simulink model "main_sim_mk15_pi"  (R2024b)
settings: Solver=ode23t  StartTime=0.0  StopTime=0.9  MaxStep=1e-7  RelTol=0.5e-5
InitFcn:
  | sw_freq=50e3;
  | kp=0.035;
  | ki=3.2;
libraries: spsSeriesRLCBranchLib x24, spsMeanLib x13, spsCurrentMeasurementLib x7, spsVoltageMeasurementLib x6, spsDiodeLib x6, spsControlledCurrentSourceLib x5, spsControlledVoltageSourceLib x5, spsMosfetLib x4, spsIdealSwitchLib x4, eeStairGenerator x2, embmathops x1, spsGroundLib x1
settings Model: SimulationMode=rapid-accelerator  Creator=adamo  LastModifiedBy=adamo
settings SolverCC: AllowMultiTaskInputOutput=on  ZeroCrossAlgorithm=Adaptive  SolverResetMethod=Robust  PositivePriorityOrder=on  DecoupledContinuousIntegration=on  MinimalZcImpactIntegration=on
settings OptimizationCC: ReuseModelBlockBuffer=off  SimCompilerOptimization=on
settings DebuggingCC: AlgebraicLoopMsg=none  MaskedZcDiagnostic=none  IgnoredZcDiagnostic=none
settings HardwareCC: ProdHWDeviceType=AMD->x86-64 (Windows64)
settings ModelReferenceCC: EnableParallelModelReferenceBuilds=on  ParallelModelReferenceMATLABWorkerInit=Copy Base Workspace  ModelReferenceMinAlgLoopOccurrences=on
settings SFSimCC: SimHardwareAcceleration=native  SimTargetLang=C++
settings RTWCC: BuildConfiguration=Faster Runs  GPUComputeCapability=3.5
settings GRTTargetCC: OptimizeReductions=on

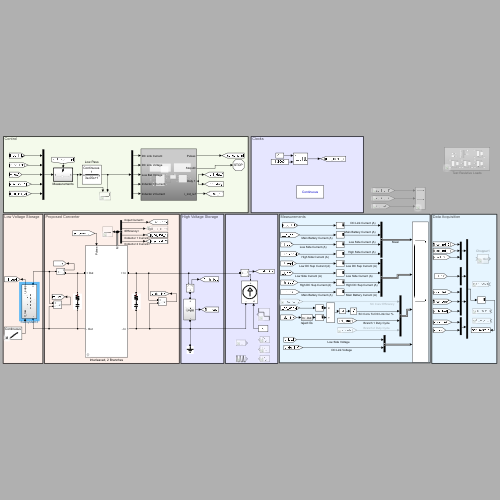
[thumbnail: Simulink's stored preview of the top-level diagram]
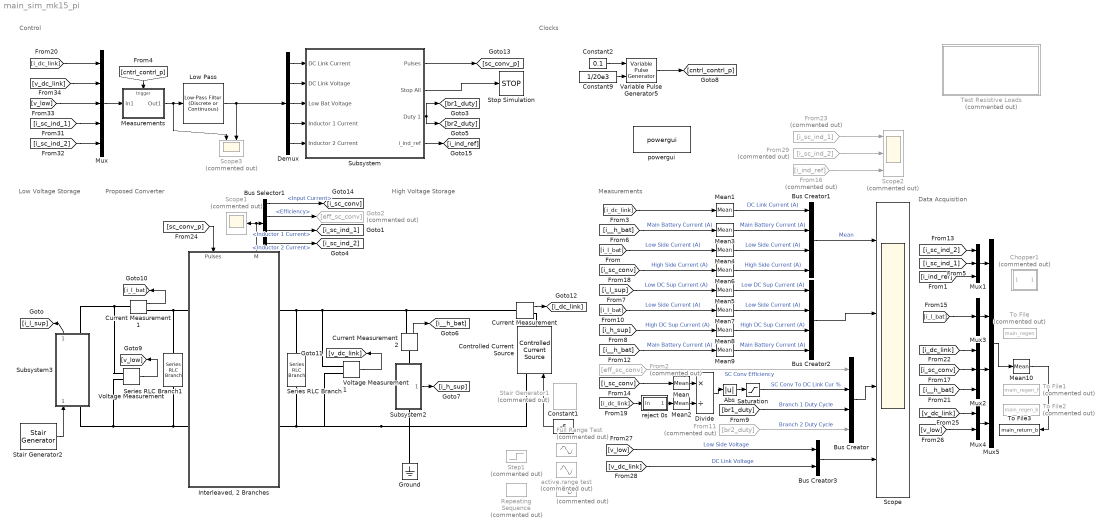
== system main_sim_mk15_pi ==
  note: Data Acquisition
  note: High Voltage Storage
  note: Low Voltage Storage
  note: Proposed Converter
  note: Clocks
  note: Control
  note: Measurements
  " " : Sin  Commented=on  Amplitude=8  Bias=18  Frequency=314.1592/10  SampleTime=0
  Abs : Abs  SaturateOnIntegerOverflow=off
  Bus Creator : BusCreator  Inputs=4
  Bus Creator1 : BusCreator  Inputs=4
  Bus Creator2 : BusCreator  Inputs=4
  Bus Creator3 : BusCreator  Inputs=2
  Bus Selector1 : BusSelector  OutputSignals=Input Current,Efficiency,Inductor 1 Current,Inductor 2 Current
  Chopper1 : Subsystem  Commented=on
  Constant1 : Constant  Value=-6
  Constant2 : Constant  Value=0.1
  Constant9 : Constant  Value=1/20e3
  Controlled Current Source : spsControlledCurrentSourceLib/Controlled Current Source  Initialize=on  Source_Type=DC  Amplitude=0  Phase=0  Frequency=0  Measurements=None
  Current Measurement : spsCurrentMeasurementLib/Current Measurement  PhasorSimulation=off  OutputType=Complex  PSBequivalent=0
  Current Measurement1 : spsCurrentMeasurementLib/Current Measurement  PhasorSimulation=off  OutputType=Complex  PSBequivalent=0
  Current Measurement2 : spsCurrentMeasurementLib/Current Measurement  PhasorSimulation=off  OutputType=Complex  PSBequivalent=0
  Demux : Demux  Outputs=5
  Divide : Product  Inputs=*/
  From11 : From  Commented=on  GotoTag=br2_duty
  From16 : From  Commented=on  GotoTag=i_ind_ref
  From2 : From  Commented=on  GotoTag=eff_sc_conv
  From23 : From  Commented=on  GotoTag=i_sc_ind_1
  From29 : From  Commented=on  GotoTag=i_sc_ind_2
  Full Range Test : Sin  Commented=on  Amplitude=52  Frequency=314.1592/8  SampleTime=0
  Goto2 : Goto  Commented=on  GotoTag=eff_sc_conv
  Ground : spsGroundLib/Ground  LConnTagsString=a
  "Interleaved, 2 Branches" : Subsystem  mask{sw_freq_mean=sw_freq, ind_ind=200e-6, fet_res_on=10e-3, bd_d_for_volt=1.1}
      mask prompts: sw_freq_mean "Switching Frequency (Hz)"; ind_ind "Branch Inductor Inductance (H)"; fet_res_on "Drain-to-Source On-Resistance (Ohm)"; bd_d_for_volt "Body Diode Forward Voltage (V)"
      settings: PortSchema="{\"entries\":[{\"content\":{\"sides\":[{\"content\":{\"connectorIds\":[\"LConn1\",\"LConn2\"]},\"type\":\"ConnectorPlacement.EquallySpacedRectSide\",\"uuid\":\"57763a22-817d-4d04-a19a-6b084199baa7\"},{\"content\":{\"connectorIds\":[\"RConn1\",\"RConn2\"],\"side\":\"RIGHT\"},\"type\":\"ConnectorPlacement.EquallySpacedRectSide\",\"uuid\":\"e5f04f53-fac9-409a-ac58-f518a07f7aa1\"},{\"content\":{\"connectorIds\":[\"In1\",\"Out1\"],\"side\":\"TOP\"},\"type\":\"ConnectorPlacement.EquallySpacedRectSide\",\"uuid\":\"7683f119-33ed-4468-84c8-2aaaca937041\"}]},\"type\":\"ConnectorPlacement.EquallySpacedConnector\",\"uuid\":\"94c2a178-e796-4540-a87e-c79e0224e730\"}],\"packageUris\":[\"http://schema.mathworks.com/mf0/Connector/R2020b\"],\"version\":\"1.0\"}"
      mask DialogControl DescTextVar Prompt: %<MaskDescription>This block impements a Two Phase Interleaved Bidirectional DC-DC Buck/Boost Converter. Input is the left side (High Voltage Side). All MOSFETs share the same characteristics.
      mask DialogControl ParameterGroupVar Prompt: Circuit Parameters
      mask DialogControl Container3 Prompt: MOSFET Parameters
  Low Pass : eeGeneralControl/Low-Pass Filter (Discrete or Continuous)  K=1  T=0.00003  B=150  A=-150  init_option=Inherited from block input  x0=0  Ts=0
  Mean : spsMeanLib/Mean  Freq=50e3/100  Vinit=0  Ts=0
  Mean{1,3..9} (8 alike) : spsMeanLib/Mean  Freq=50e3/50  Vinit=0  Ts=0
  Mean10 : spsMeanLib/Mean  Freq=50e3/100  Vinit=0  Ts=0
  Mean2 : spsMeanLib/Mean  Freq=50e3/100  Vinit=0  Ts=0
  Measurements : Subsystem  TreatAsAtomicUnit=on
  Mux : Mux  Inputs=5
  Mux1 : Mux  Inputs=3
  Mux2 : Mux  Inputs=3
  Mux3 : Mux  Inputs=1
  Mux4 : Mux  Inputs=2
  Mux5 : Mux
  Repeating Sequence : simulink/Sources/Repeating Sequence  Commented=on  rep_seq_t=[0 0.5 1 2]*2  rep_seq_y=[0 16 0 0]
  Saturation : Saturate  UpperLimit=1  LowerLimit=0
  Scope : Scope  NumInputPorts=4
  Scope1 : Scope  Commented=on
  Scope2 : Scope  Commented=on  NumInputPorts=3
  Scope3 : Scope  Commented=on  NumInputPorts=2
  Series RLC Branch : spsSeriesRLCBranchLib/Series RLC Branch  LConnTagsString=__new0  RConnTagsString=__new0  BranchType=RC  Resistance=1e-4  Inductance=1e-3  SetiL0=off  InitialCurrent=0  Capacitance=800e-6  Setx0=on  InitialVoltage=80  Measurements=None
  Series RLC Branch1 : spsSeriesRLCBranchLib/Series RLC Branch  LConnTagsString=__new0  RConnTagsString=__new0  BranchType=RC  Resistance=1e-4  Inductance=1e-3  SetiL0=off  InitialCurrent=0  Capacitance=400e-6  Setx0=on  InitialVoltage=15  Measurements=None
  Stair Generator1 : spsStairGeneratorLib/Stair Generator  Commented=on  t=[0:1:3]  e=[12.5:-2.5:5]  Ts=0
  Stair Generator2 : eeStairGenerator/Stair Generator  LabelModeActiveChoice=Continuous  TimeInput=[0:0.15:1]  AmplitudeInput=[15:5:45]  SampleTime=0  RepeatPattern=off  OutDataTypeStr=double
      settings: LibrarySourceBlock=ee_sl_lib/General Control/Stair Generator
  Step1 : Step  Commented=on  Time=0.1  Before=27  After=-25  SampleTime=0
  Stop Simulation : Stop
  Subsystem : Subsystem
  Subsystem2 : Subsystem
      settings: PortSchema="{\"entries\":[{\"content\":{\"sides\":[{\"content\":{},\"type\":\"ConnectorPlacement.EquallySpacedRectSide\",\"uuid\":\"89586188-a7fa-42d8-902c-41f5e85746df\"},{\"content\":{\"connectorIds\":[\"Out1\"],\"side\":\"RIGHT\"},\"type\":\"ConnectorPlacement.EquallySpacedRectSide\",\"uuid\":\"d8c02237-7822-43ca-9dbf-595cafdf61ba\"},{\"content\":{\"connectorIds\":[\"LConn1\"],\"side\":\"TOP\"},\"type\":\"ConnectorPlacement.EquallySpacedRectSide\",\"uuid\":\"69757e4c-b908-4056-b98e-0c667e12b99a\"},{\"content\":{\"connectorIds\":[\"RConn1\"],\"side\":\"BOTTOM\"},\"type\":\"ConnectorPlacement.EquallySpacedRectSide\",\"uuid\":\"ccf2e3d8-e338-404e-98cd-f765717e085e\"}]},\"type\":\"ConnectorPlacement.EquallySpacedConnector\",\"uuid\":\"a290fee4-a270-4f54-b8a3-7452b5039597\"}],\"packageUris\":[\"http://schema.mathworks.com/mf0/Connector/R2020b\"],\"version\":\"1.0\"}"
  Subsystem3 : Subsystem
      settings: PortSchema="{\"entries\":[{\"content\":{\"sides\":[{\"content\":{},\"type\":\"ConnectorPlacement.EquallySpacedRectSide\",\"uuid\":\"89586188-a7fa-42d8-902c-41f5e85746df\"},{\"content\":{\"side\":\"RIGHT\"},\"type\":\"ConnectorPlacement.EquallySpacedRectSide\",\"uuid\":\"d8c02237-7822-43ca-9dbf-595cafdf61ba\"},{\"content\":{\"connectorIds\":[\"LConn1\",\"Out1\"],\"side\":\"TOP\"},\"type\":\"ConnectorPlacement.EquallySpacedRectSide\",\"uuid\":\"69757e4c-b908-4056-b98e-0c667e12b99a\"},{\"content\":{\"connectorIds\":[\"RConn1\",\"In1\"],\"side\":\"BOTTOM\"},\"type\":\"ConnectorPlacement.EquallySpacedRectSide\",\"uuid\":\"e30ca493-d5d4-4c79-9ea0-2752edd701ef\"}]},\"type\":\"ConnectorPlacement.EquallySpacedConnector\",\"uuid\":\"a290fee4-a270-4f54-b8a3-7452b5039597\"}],\"packageUris\":[\"http://schema.mathworks.com/mf0/Connector/R2020b\"],\"version\":\"1.0\"}"
  Test Resistive Loads : Subsystem  Commented=on
  To File : ToFile  Commented=on  Filename=main_regen
  To File1 : ToFile  Commented=on  Filename=main_regen_f
  To File2 : ToFile  Commented=on  Filename=main_regen_b
  To File3 : ToFile  Filename=main_return_b
  Variable Pulse Generator5 : VariablePulseGenerator  AllowZeroPulseWidth=on  SampleTime=0.1
  Voltage Measurement : spsVoltageMeasurementLib/Voltage Measurement  PhasorSimulation=off  OutputType=Complex  PSBequivalent=0
  Voltage Measurement1 : spsVoltageMeasurementLib/Voltage Measurement  PhasorSimulation=off  OutputType=Complex  PSBequivalent=0
  active range test : Sin  Commented=on  Amplitude=24  Bias=4  Frequency=314.1592/32  SampleTime=0
  powergui : spspowerguiLib/powergui  Priority=1  SimulationMode=Continuous  SampleTime=50e-6  frequency=60  Iterations=50  frequencyindice=0  Pbase=100e6  ErrMax=1e-4  UnitsV=kV  UnitsW=MW  buscounter=0  FunctionMessages=off  echomessages=off  EnableUseOfTLC=off  CurrentSourceSwitches=off  DisableSnubberDevices=on  DisableRonSwitches=off  DisableVfSwitches=off  DisplayEquations=off  AutomaticDiscreteSolvers=off  SolverType=Tustin/Backward Euler (TBE)  Interpol=off  ExternalGateDelay=off  methode=off  Ts=100  x0status=blocks  SPID=on  SwTol=0  HookPort=off  NonlinearTolerance=1e-4  nMaxIteration=100  ContinueOnMaxIteration=off  RestoreLinks=warning  ResistiveCurrentMeasurement=off  Frange=[0:2:500]  Ylog=off  Xlog=on  ShowGrid=off  save=off  variable=ZData  structure=0  ZoomFFT=off  StartTime=0.0  cycles=1  DisplayStyle=1  fundamental=60  FreqAxis=off  MaxFrequency=1000  frequencyindicesteady=1  RmsSteady=1  display=off
  reject 0s : Subsystem
  wires:
  Bus Creator2/1 -> Scope/2
  Mean3/1 -> Bus Creator1/2  "Main Battery Current (A)"
  Mean4/1 -> Bus Creator1/3  "Low Side Current (A)"
  Bus Selector1/2 -> Goto2/1  "<Efficiency>"
  From2/1 -> Bus Creator/1  "SC Conv Efficiency"
  Bus Selector1/1 -> [i_sc_conv]  "<Input Current>"
  reject 0s/1(Out) -> Mean2/1
  Divide/1 -> Abs/1
  Abs/1 -> Saturation/1
  [i_sc_conv] -> Mean/1
  Saturation/1 -> Bus Creator/2  "SC Conv To DC Link Cur %"
  [i_dc_link] -> reject 0s/1(In)
  Bus Creator/1 -> Scope/3
  Bus Creator1/1 -> Scope/1  "Mean"
  Mean/1 -> Divide/1
  Mean2/1 -> Divide/2
  Mean1/1 -> Bus Creator1/1  "DC Link Current (A)"
  [i__h_bat] -> Mean3/1  "Main Battery Current (A)"
  [i_l_bat] -> Mean4/1  "Low Side Current (A)"
  Mean6/1 -> Bus Creator1/4  "High Side Current (A)"
  [i_sc_conv] -> Mean6/1  "High Side Current (A)"
  [sc_conv_p] -> "Interleaved, 2 Branches"/1(Pulses)
  Subsystem2/1(i_supp) -> [i_h_sup]
  [i_dc_link] -> Mean1/1
  Current Measurement/1 -> [i_dc_link]
  Bus Selector1/3 -> [i_sc_ind_1]  "<Inductor 1 Current>"
  Bus Selector1/4 -> [i_sc_ind_2]  "<Inductor 2 Current>"
  Voltage Measurement/1 -> [v_low]
  Current Measurement1/1 -> [i_l_bat]
  Constant2/1 -> Variable Pulse Generator5/1
  Constant9/1 -> Variable Pulse Generator5/2
  Variable Pulse Generator5/1 -> [cntrl_contrl_p]
  Subsystem/1(Pulses) -> [sc_conv_p]
  [i_sc_ind_2] -> Mux/5
  [i_sc_ind_1] -> Mux/4
  [v_low] -> Mux/3
  [v_dc_link] -> Mux/2
  [i_dc_link] -> Mux/1
  Demux/1 -> Subsystem/1(DC Link Current)
  Demux/2 -> Subsystem/2(DC Link Voltage)
  Demux/3 -> Subsystem/3(Low Bat Voltage)
  Demux/5 -> Subsystem/5(Inductor 2 Current)
  Demux/4 -> Subsystem/4(Inductor 1 Current)
  [cntrl_contrl_p] -> Measurements/Trigger
  Subsystem/2(Stop All) -> Stop Simulation/1
  Subsystem/3(Duty 1) -> [br1_duty], [br2_duty]
  From11/1 -> Bus Creator/4  "Branch 2 Duty Cycle"
  [br1_duty] -> Bus Creator/3  "Branch 1 Duty Cycle"
  Bus Creator3/1 -> Scope/4
  Current Measurement2/1 -> [i__h_bat]
  Subsystem3/1(i_supp) -> [i_l_sup]
  Mean5/1 -> Bus Creator2/1  "Low DC Sup Current (A)"
  Mean7/1 -> Bus Creator2/2  "Low Side Current (A)"
  Mean8/1 -> Bus Creator2/3  "High DC Sup Current (A)"
  Mean9/1 -> Bus Creator2/4  "Main Battery Current (A)"
  [i_l_sup] -> Mean5/1  "Low DC Sup Current (A)"
  [i_l_bat] -> Mean7/1  "Low Side Current (A)"
  [i_h_sup] -> Mean8/1  "High DC Sup Current (A)"
  [i__h_bat] -> Mean9/1  "Main Battery Current (A)"
  Voltage Measurement1/1 -> [v_dc_link]
  Mux/1 -> Measurements/1(In1)
  Measurements/1(Out1) -> Scope3/1, Low Pass/1
  Subsystem/4(i_ind_ref) -> [i_ind_ref]
  [i_sc_ind_2] -> Mux1/1
  [i_sc_ind_1] -> Mux1/2
  [i_ind_ref] -> Mux1/3
  [i_dc_link] -> Mux2/1
  [i_sc_conv] -> Mux2/2
  [i__h_bat] -> Mux2/3
  [i_l_bat] -> Mux3/1
  [v_low] -> Mux4/2
  [v_dc_link] -> Mux4/1
  Mux1/1 -> Mux5/1
  Mux3/1 -> Mux5/2
  Mux2/1 -> Mux5/3
  Mux4/1 -> Mux5/4
  Mux5/1 -> Mean10/1
  Stair Generator2/1 -> Subsystem3/1(V_low)
  [v_low] -> Bus Creator3/1  "Low Side Voltage"
  [v_dc_link] -> Bus Creator3/2  "DC Link Voltage"
  "Interleaved, 2 Branches"/1(M) -> Scope1/1, Bus Selector1/1
  Low Pass/1 -> Demux/1, Scope3/2
  Constant1/1 -> Controlled Current Source/1
  Mean10/1 -> To File3/1
  From23/1 -> Scope2/1
  From16/1 -> Scope2/3
  From29/1 -> Scope2/2
  connections:
  Series RLC Branch/RConn1 -- Voltage Measurement1/LConn2 -- Controlled Current Source/LConn1 -- Ground/LConn1 -- Subsystem2/RConn1 -- "Interleaved, 2 Branches"/RConn2
  "Interleaved, 2 Branches"/LConn2 -- Series RLC Branch1/RConn1 -- Subsystem3/RConn1 -- Voltage Measurement/LConn2
  Controlled Current Source/RConn1 -- Current Measurement/RConn1
  Voltage Measurement/LConn1 -- Subsystem3/LConn1 -- Current Measurement1/LConn1
  Current Measurement/LConn1 -- Current Measurement2/RConn1 -- Voltage Measurement1/LConn1 -- "Interleaved, 2 Branches"/RConn1 -- Series RLC Branch/LConn1
  "Interleaved, 2 Branches"/LConn1 -- Series RLC Branch1/LConn1 -- Current Measurement1/RConn1
  Current Measurement2/LConn1 -- Subsystem2/LConn1

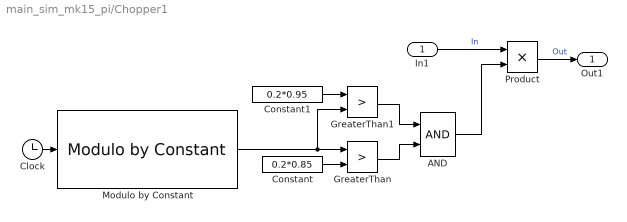
== system main_sim_mk15_pi/Chopper1 ==
  In1 : Inport
  AND : Logic  IconShape=distinctive  AllPortsSameDT=off  OutDataTypeStr=boolean
  Clock : Clock
  Constant : Constant  Value=0.2*0.85
  Constant1 : Constant  Value=0.2*0.95
  GreaterThan : RelationalOperator  Operator=>  OutDataTypeStr=boolean  RndMeth=Simplest  InputSameDT=off
  GreaterThan1 : RelationalOperator  Operator=>  OutDataTypeStr=boolean  RndMeth=Simplest  InputSameDT=off
  Modulo by Constant : embmathops/Modulo by Constant  Denominator=0.2  SimulateUsing=Code generation
  Product : Product
  Out1 : Outport
  wires:
  Clock/1 -> Modulo by Constant/1
  Constant/1 -> GreaterThan/2
  GreaterThan1/1 -> AND/1
  GreaterThan/1 -> AND/2
  AND/1 -> Product/2
  Modulo by Constant/1 -> GreaterThan1/2, GreaterThan/1
  Constant1/1 -> GreaterThan1/1
  In1/1 -> Product/1  "In"
  Product/1 -> Out1/1  "Out"

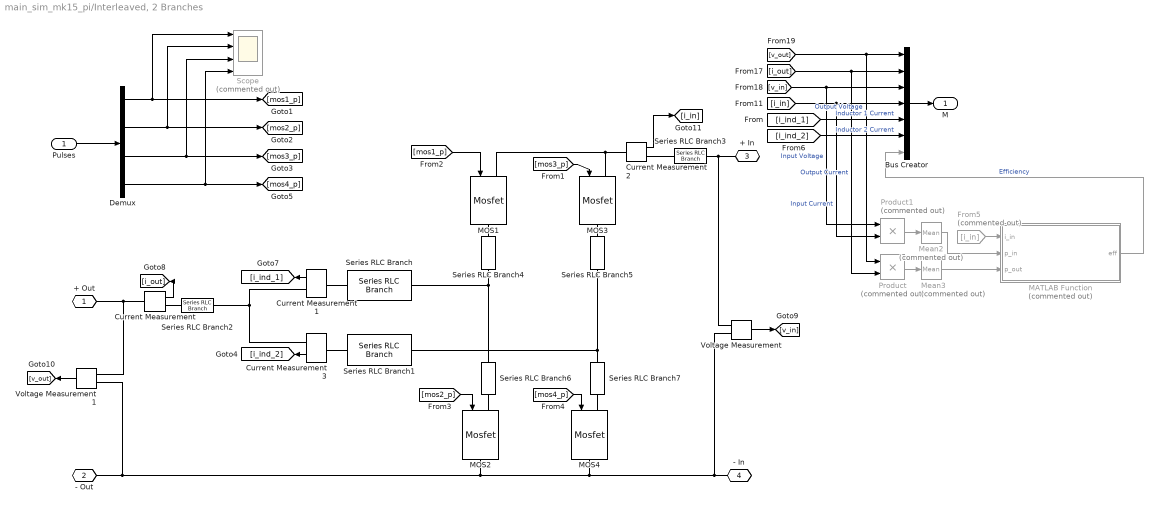
== system main_sim_mk15_pi/Interleaved, 2 Branches ==
  Pulses : Inport
  Bus Creator : BusCreator  Inputs=7
  Current Measurement{,1..3} (4 alike) : spsCurrentMeasurementLib/Current Measurement  PhasorSimulation=off  OutputType=Complex  PSBequivalent=0
  Demux : Demux
  From5 : From  Commented=on  GotoTag=i_in
  MATLAB Function : MATLAB Function  Commented=on  TreatAsAtomicUnit=on
  MOS{1..4} (4 alike) : spsMosfetLib/Mosfet  Ron=fet_res_on  Lon=0  Rd=0.01  Vfd=bd_d_for_volt  IC=0  Rs=1e5  Cs=inf  Measurements=off
  Mean2 : spsMeanLib/Mean  Commented=on  Freq=sw_freq_mean/10  Vinit=0  Ts=0
  Mean3 : spsMeanLib/Mean  Commented=on  Freq=sw_freq_mean/10  Vinit=0  Ts=0
  Product : Product  Commented=on
  Product1 : Product  Commented=on
  Scope : Scope  Commented=on  NumInputPorts=4
  Series RLC Branch : spsSeriesRLCBranchLib/Series RLC Branch  LConnTagsString=__new0  RConnTagsString=__new0  BranchType=RL  Resistance=1e-3  Inductance=ind_ind  SetiL0=off  InitialCurrent=1e-3  Capacitance=1e-6  Setx0=off  InitialVoltage=0  Measurements=None
  Series RLC Branch1 : spsSeriesRLCBranchLib/Series RLC Branch  LConnTagsString=__new0  RConnTagsString=__new0  BranchType=RL  Resistance=1e-3  Inductance=ind_ind  SetiL0=off  InitialCurrent=1e-3  Capacitance=1e-6  Setx0=off  InitialVoltage=0  Measurements=None
  Series RLC Branch2 : spsSeriesRLCBranchLib/Series RLC Branch  LConnTagsString=__new0  RConnTagsString=__new0  BranchType=R  Resistance=5e-3  Inductance=5e-4  SetiL0=off  InitialCurrent=1e-3  Capacitance=1e-6  Setx0=off  InitialVoltage=0  Measurements=None
  Series RLC Branch3 : spsSeriesRLCBranchLib/Series RLC Branch  LConnTagsString=__new0  RConnTagsString=__new0  BranchType=R  Resistance=5e-3  Inductance=5e-4  SetiL0=off  InitialCurrent=1e-3  Capacitance=1e-6  Setx0=off  InitialVoltage=0  Measurements=None
  Series RLC Branch{4..7} (4 alike) : spsSeriesRLCBranchLib/Series RLC Branch  LConnTagsString=__new0  RConnTagsString=__new0  BranchType=R  Resistance=1e-3  Inductance=5e-4  SetiL0=off  InitialCurrent=1e-3  Capacitance=1e-6  Setx0=off  InitialVoltage=0  Measurements=None
  Voltage Measurement : spsVoltageMeasurementLib/Voltage Measurement  PhasorSimulation=off  OutputType=Complex  PSBequivalent=0
  Voltage Measurement1 : spsVoltageMeasurementLib/Voltage Measurement  PhasorSimulation=off  OutputType=Complex  PSBequivalent=0
  + Out : PMIOPort  Side=Left
  - Out : PMIOPort  Port=2  Side=Left
  "+ In " : PMIOPort  Port=3  Side=Right
  "- In " : PMIOPort  Port=4  Side=Right
  M : Outport
  wires:
  [mos1_p] -> MOS1/1
  [mos2_p] -> MOS2/1
  Current Measurement1/1 -> [i_ind_1]
  Current Measurement2/1 -> [i_in]
  Voltage Measurement1/1 -> [v_out]
  Voltage Measurement/1 -> [v_in]
  [i_ind_2] -> Bus Creator/6  "Inductor 2 Current"
  Bus Creator/1 -> M/1
  [v_in] -> Bus Creator/3, Product1/1  "Input Voltage"
  [i_out] -> Product/2, Bus Creator/2  "Output Current"
  [i_in] -> Product1/2, Bus Creator/4  "Input Current"
  [v_out] -> Product/1, Bus Creator/1  "Output Voltage"
  MATLAB Function/1(eff) -> Bus Creator/7  "Efficiency"
  Product/1 -> Mean3/1
  Product1/1 -> Mean2/1
  From5/1 -> MATLAB Function/1(i_in)
  Pulses/1 -> Demux/1
  Demux/1 -> Scope/1, [mos1_p]
  Mean2/1 -> MATLAB Function/2(p_in)
  Mean3/1 -> MATLAB Function/3(p_out)
  Current Measurement/1 -> [i_out]
  [mos3_p] -> MOS3/1
  Current Measurement3/1 -> [i_ind_2]
  [i_ind_1] -> Bus Creator/5  "Inductor 1 Current"
  Demux/3 -> Scope/3, [mos3_p]
  Demux/4 -> Scope/4, [mos4_p]
  Demux/2 -> Scope/2, [mos2_p]
  [mos4_p] -> MOS4/1
  connections:
  MOS1/LConn1 -- Current Measurement2/LConn1 -- MOS3/LConn1
  Voltage Measurement1/LConn1 -- Current Measurement/LConn1 -- + Out/RConn1
  "+ In "/RConn1 -- Voltage Measurement/LConn1 -- Series RLC Branch3/RConn1
  "- In "/RConn1 -- Voltage Measurement/LConn2 -- Voltage Measurement1/LConn2 -- - Out/RConn1 -- MOS2/RConn1 -- MOS4/RConn1
  Series RLC Branch/LConn1 -- Current Measurement1/LConn1
  Series RLC Branch/RConn1 -- Series RLC Branch6/LConn1 -- Series RLC Branch4/RConn1
  Series RLC Branch1/RConn1 -- Series RLC Branch7/LConn1 -- Series RLC Branch5/RConn1
  Series RLC Branch1/LConn1 -- Current Measurement3/LConn1
  Series RLC Branch2/RConn1 -- Current Measurement3/RConn1 -- Current Measurement1/RConn1
  Series RLC Branch2/LConn1 -- Current Measurement/RConn1
  Series RLC Branch4/LConn1 -- MOS1/RConn1
  Series RLC Branch5/LConn1 -- MOS3/RConn1
  Series RLC Branch6/RConn1 -- MOS2/LConn1
  Series RLC Branch7/RConn1 -- MOS4/LConn1
  Series RLC Branch3/LConn1 -- Current Measurement2/RConn1

== system main_sim_mk15_pi/Measurements ==
  In1 : Inport
  Trigger : TriggerPort  VariantControl=(inherit)
  Zero-Order Hold : ZeroOrderHold  SampleTime=-1
  Out1 : Outport
  wires:
  In1/1 -> Zero-Order Hold/1
  Zero-Order Hold/1 -> Out1/1

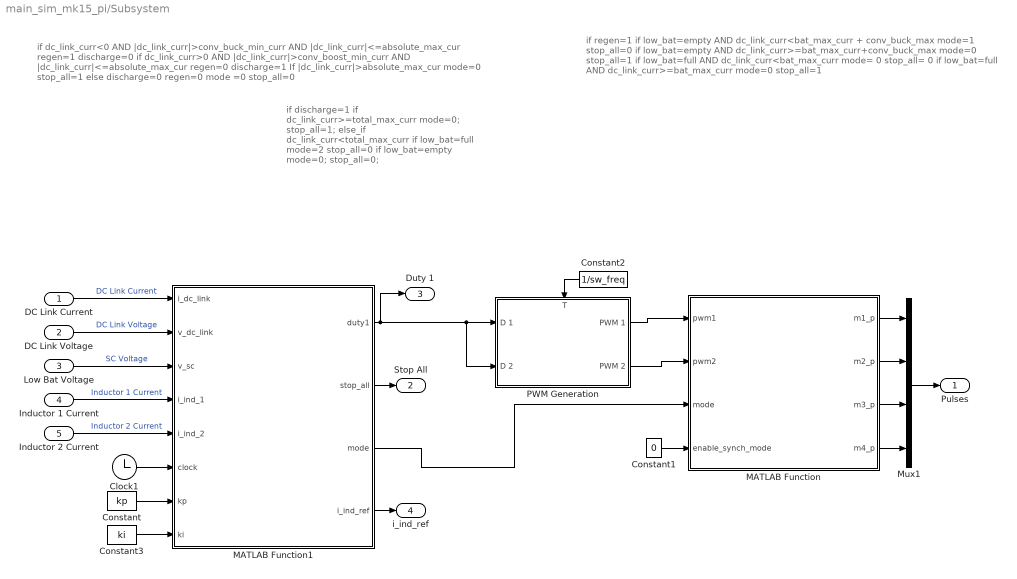
== system main_sim_mk15_pi/Subsystem ==
  note: if regen=1
      | 	if low_bat=empty AND dc_link_curr<bat_max_curr + conv_buck_max
      | 		mode=1
      | 		stop_all=0
      | 	if low_bat=empty AND dc_link_curr>=bat_max_curr+conv_buck_max
      | 		mode=0
      | 		stop_all=1
      | 	if low_bat=full AND dc_link_curr<bat_max_curr
      | 		mode= 0
      | 		stop_all= 0
      | 	if low_bat=full AND dc_link_curr>=bat_max_curr
      | 		mode=0
      | 		stop_all=1
  note: if discharge=1
      | 	if dc_link_curr>=total_max_curr
      | 		mode=0;
      | 		stop_all=1;
      | 	else_if dc_link_curr<total_max_curr
      | 		if low_bat=full
      | 			mode=2
      | 			stop_all=0
      | 		if low_bat=empty
      | 			mode=0;
      | 			stop_all=0;
  note: if dc_link_curr<0 AND |dc_link_curr|>conv_buck_min_curr AND |dc_link_curr|<=absolute_max_cur
      | 	regen=1
      | 	discharge=0
      | if dc_link_curr>0 AND |dc_link_curr|>conv_boost_min_curr AND |dc_link_curr|<=absolute_max_cur
      | 	regen=0
      | 	discharge=1
      | If  |dc_link_curr|>absolute_max_cur
      | 	mode=0
      | 	stop_all=1
      | else
      | 	discharge=0
      | 	regen=0
      | 	mode =0
      | 	stop_all=0
  DC Link Current : Inport
  DC Link Voltage : Inport  Port=2
  Low Bat Voltage : Inport  Port=3
  Inductor 1 Current : Inport  Port=4
  Inductor 2 Current : Inport  Port=5
  Clock1 : Clock
      settings: Decimation=20
  Constant : Constant  Value=kp
  Constant1 : Constant  Value=0
  Constant2 : Constant  Value=1/sw_freq
  Constant3 : Constant  Value=ki
  MATLAB Function : MATLAB Function  TreatAsAtomicUnit=on
  MATLAB Function1 : MATLAB Function  TreatAsAtomicUnit=on
  Mux1 : Mux
  PWM Generation : Subsystem
      settings: PortSchema="{\"entries\":[{\"content\":{\"sides\":[{\"content\":{\"connectorIds\":[\"In1\",\"In2\"]},\"type\":\"ConnectorPlacement.EquallySpacedRectSide\",\"uuid\":\"83f7ddc5-a76f-4bd9-b3c1-9fd524e2bc79\"},{\"content\":{\"connectorIds\":[\"Out1\",\"Out2\"],\"side\":\"RIGHT\"},\"type\":\"ConnectorPlacement.EquallySpacedRectSide\",\"uuid\":\"761d98eb-d7f1-4fa1-8255-54b7e6584824\"},{\"content\":{\"connectorIds\":[\"In3\"],\"side\":\"TOP\"},\"type\":\"ConnectorPlacement.EquallySpacedRectSide\",\"uuid\":\"fcf92395-65ef-4712-95c3-1cc1de5b2992\"}]},\"type\":\"ConnectorPlacement.EquallySpacedConnector\",\"uuid\":\"c82b4b62-fa36-4445-aa1a-cfaf75c093b5\"}],\"packageUris\":[\"http://schema.mathworks.com/mf0/Connector/R2020b\"],\"version\":\"1.0\"}"
  Pulses : Outport
  Stop All : Outport  Port=2
  Duty 1 : Outport  Port=3
  i_ind_ref : Outport  Port=4
  wires:
  DC Link Voltage/1 -> MATLAB Function1/2(v_dc_link)  "DC Link Voltage"
  DC Link Current/1 -> MATLAB Function1/1(i_dc_link)  "DC Link Current"
  Low Bat Voltage/1 -> MATLAB Function1/3(v_sc)  "SC Voltage"
  Inductor 1 Current/1 -> MATLAB Function1/4(i_ind_1)  "Inductor 1 Current"
  Inductor 2 Current/1 -> MATLAB Function1/5(i_ind_2)  "Inductor 2 Current"
  MATLAB Function1/2(stop_all) -> Stop All/1
  MATLAB Function1/3(mode) -> MATLAB Function/3(mode)
  Mux1/1 -> Pulses/1
  Clock1/1 -> MATLAB Function1/6(clock)
  MATLAB Function/1(m1_p) -> Mux1/1
  MATLAB Function/2(m2_p) -> Mux1/2
  MATLAB Function/3(m3_p) -> Mux1/3
  MATLAB Function/4(m4_p) -> Mux1/4
  Constant1/1 -> MATLAB Function/4(enable_synch_mode)
  MATLAB Function1/1(duty1) -> Duty 1/1, PWM Generation/2(D 2), PWM Generation/1(D 1)
  PWM Generation/1(PWM 1) -> MATLAB Function/1(pwm1)
  PWM Generation/2(PWM 2) -> MATLAB Function/2(pwm2)
  Constant2/1 -> PWM Generation/3(T)
  MATLAB Function1/4(i_ind_ref) -> i_ind_ref/1
  Constant/1 -> MATLAB Function1/7(kp)
  Constant3/1 -> MATLAB Function1/8(ki)

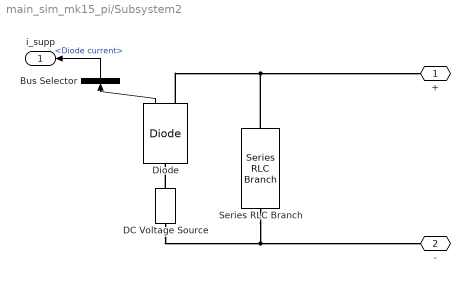
== system main_sim_mk15_pi/Subsystem2 ==
  Bus Selector : BusSelector  OutputSignals=Diode current
  DC Voltage Source : spsDCVoltageSourceLib/DC Voltage Source  Amplitude=80  Measurements=None
  Diode : spsDiodeLib/Diode  Ron=0.001  Lon=0  Vf=0.01  IC=0  UseSnubber=0  Rs=500  Cs=250e-9  Measurements=on
  Series RLC Branch : spsSeriesRLCBranchLib/Series RLC Branch  LConnTagsString=__new0  RConnTagsString=__new0  BranchType=R  Resistance=6.4  Inductance=1e-3  SetiL0=off  InitialCurrent=0  Capacitance=1e-6  Setx0=off  InitialVoltage=0  Measurements=None
  + : PMIOPort  Side=Left
  - : PMIOPort  Port=2  Side=Right
  i_supp : Outport
  wires:
  Diode/1 -> Bus Selector/1
  Bus Selector/1 -> i_supp/1  "<Diode current>"
  connections:
  Series RLC Branch/LConn1 -- +/RConn1 -- Diode/RConn1
  Series RLC Branch/RConn1 -- -/RConn1 -- DC Voltage Source/LConn1
  DC Voltage Source/RConn1 -- Diode/LConn1

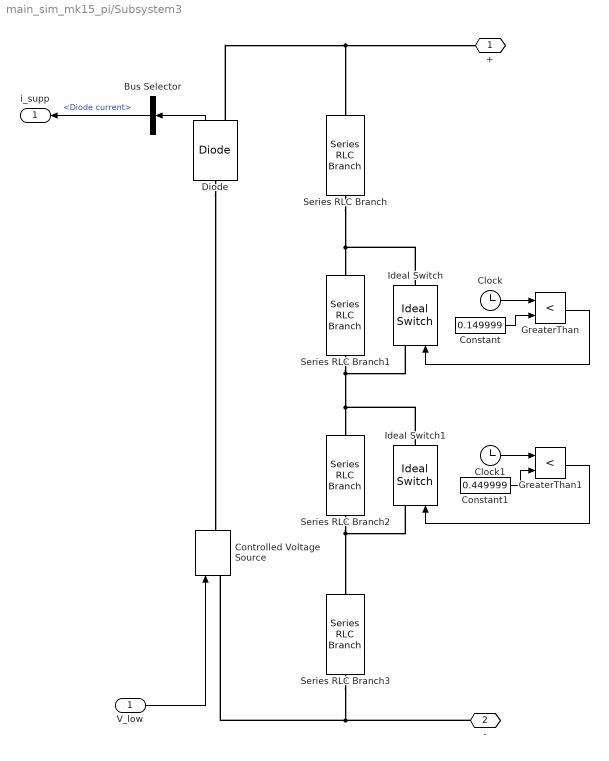
== system main_sim_mk15_pi/Subsystem3 ==
  V_low : Inport
  Bus Selector : BusSelector  OutputSignals=Diode current
  Clock : Clock
  Clock1 : Clock
  Constant : Constant  Value=0.149999
  Constant1 : Constant  Value=0.449999
  Controlled Voltage Source : spsControlledVoltageSourceLib/Controlled Voltage Source  Initialize=on  Source_Type=DC  Amplitude=40  Phase=0  Frequency=0  Measurements=None
  Diode : spsDiodeLib/Diode  Ron=0.001  Lon=0  Vf=0.01  IC=0  UseSnubber=0  Rs=500  Cs=250e-9  Measurements=on
  GreaterThan : RelationalOperator  Operator=<  OutDataTypeStr=boolean  RndMeth=Simplest  InputSameDT=off
  GreaterThan1 : RelationalOperator  Operator=<  OutDataTypeStr=boolean  RndMeth=Simplest  InputSameDT=off
  Ideal Switch : spsIdealSwitchLib/Ideal Switch  Ron=0.001  Lon=0  IC=0  Rs=1e5  Cs=inf  Measurements=off
  Ideal Switch1 : spsIdealSwitchLib/Ideal Switch  Ron=0.001  Lon=0  IC=0  Rs=1e5  Cs=inf  Measurements=off
  Series RLC Branch : spsSeriesRLCBranchLib/Series RLC Branch  LConnTagsString=__new0  RConnTagsString=__new0  BranchType=R  Resistance=0.32  Inductance=1e-9  SetiL0=off  InitialCurrent=0  Capacitance=1e-6  Setx0=off  InitialVoltage=0  Measurements=None
  Series RLC Branch1 : spsSeriesRLCBranchLib/Series RLC Branch  LConnTagsString=__new0  RConnTagsString=__new0  BranchType=R  Resistance=0.33  Inductance=1e-3  SetiL0=off  InitialCurrent=0  Capacitance=1e-6  Setx0=off  InitialVoltage=0  Measurements=None
  Series RLC Branch2 : spsSeriesRLCBranchLib/Series RLC Branch  LConnTagsString=__new0  RConnTagsString=__new0  BranchType=R  Resistance=0.5  Inductance=1e-3  SetiL0=off  InitialCurrent=0  Capacitance=1e-6  Setx0=off  InitialVoltage=0  Measurements=None
  Series RLC Branch3 : spsSeriesRLCBranchLib/Series RLC Branch  LConnTagsString=__new0  RConnTagsString=__new0  BranchType=R  Resistance=6.4  Inductance=1e-9  SetiL0=off  InitialCurrent=0  Capacitance=1e-6  Setx0=off  InitialVoltage=0  Measurements=None
  + : PMIOPort  Side=Left
  - : PMIOPort  Port=2  Side=Right
  i_supp : Outport
  wires:
  Diode/1 -> Bus Selector/1
  Bus Selector/1 -> i_supp/1  "<Diode current>"
  V_low/1 -> Controlled Voltage Source/1
  Clock/1 -> GreaterThan/1
  Constant/1 -> GreaterThan/2
  GreaterThan/1 -> Ideal Switch/1
  Constant1/1 -> GreaterThan1/2
  Clock1/1 -> GreaterThan1/1
  GreaterThan1/1 -> Ideal Switch1/1
  connections:
  Diode/LConn1 -- Controlled Voltage Source/RConn1
  Ideal Switch/RConn1 -- Series RLC Branch/RConn1 -- Series RLC Branch1/LConn1
  Series RLC Branch1/RConn1 -- Series RLC Branch2/LConn1 -- Ideal Switch1/RConn1 -- Ideal Switch/LConn1
  Series RLC Branch2/RConn1 -- Ideal Switch1/LConn1 -- Series RLC Branch3/LConn1
  Diode/RConn1 -- +/RConn1 -- Series RLC Branch/LConn1
  Series RLC Branch3/RConn1 -- -/RConn1 -- Controlled Voltage Source/LConn1

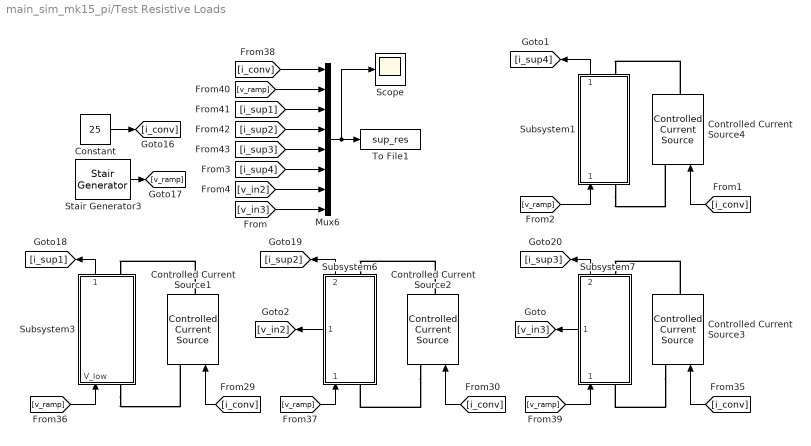
== system main_sim_mk15_pi/Test Resistive Loads ==
  Constant : Constant  Value=25
  Controlled Current Source{1..4} (4 alike) : spsControlledCurrentSourceLib/Controlled Current Source  Initialize=on  Source_Type=DC  Amplitude=0  Phase=0  Frequency=0  Measurements=None
  Mux6 : Mux  Inputs=8
  Scope : Scope
  Stair Generator3 : eeStairGenerator/Stair Generator  LabelModeActiveChoice=Continuous  TimeInput=[0:0.15:1]  AmplitudeInput=[15:5:40 40]  SampleTime=0  RepeatPattern=off  OutDataTypeStr=double
  Subsystem1 : Subsystem
      settings: PortSchema="{\"entries\":[{\"content\":{\"sides\":[{\"content\":{},\"type\":\"ConnectorPlacement.EquallySpacedRectSide\",\"uuid\":\"89586188-a7fa-42d8-902c-41f5e85746df\"},{\"content\":{\"side\":\"RIGHT\"},\"type\":\"ConnectorPlacement.EquallySpacedRectSide\",\"uuid\":\"d8c02237-7822-43ca-9dbf-595cafdf61ba\"},{\"content\":{\"connectorIds\":[\"LConn1\",\"Out1\"],\"side\":\"TOP\"},\"type\":\"ConnectorPlacement.EquallySpacedRectSide\",\"uuid\":\"69757e4c-b908-4056-b98e-0c667e12b99a\"},{\"content\":{\"connectorIds\":[\"RConn1\",\"In1\"],\"side\":\"BOTTOM\"},\"type\":\"ConnectorPlacement.EquallySpacedRectSide\",\"uuid\":\"e30ca493-d5d4-4c79-9ea0-2752edd701ef\"}]},\"type\":\"ConnectorPlacement.EquallySpacedConnector\",\"uuid\":\"a290fee4-a270-4f54-b8a3-7452b5039597\"}],\"packageUris\":[\"http://schema.mathworks.com/mf0/Connector/R2020b\"],\"version\":\"1.0\"}"
  Subsystem3 : Subsystem
      settings: PortSchema="{\"entries\":[{\"content\":{\"sides\":[{\"content\":{},\"type\":\"ConnectorPlacement.EquallySpacedRectSide\",\"uuid\":\"89586188-a7fa-42d8-902c-41f5e85746df\"},{\"content\":{\"side\":\"RIGHT\"},\"type\":\"ConnectorPlacement.EquallySpacedRectSide\",\"uuid\":\"d8c02237-7822-43ca-9dbf-595cafdf61ba\"},{\"content\":{\"connectorIds\":[\"LConn1\",\"Out1\"],\"side\":\"TOP\"},\"type\":\"ConnectorPlacement.EquallySpacedRectSide\",\"uuid\":\"69757e4c-b908-4056-b98e-0c667e12b99a\"},{\"content\":{\"connectorIds\":[\"RConn1\",\"In1\"],\"side\":\"BOTTOM\"},\"type\":\"ConnectorPlacement.EquallySpacedRectSide\",\"uuid\":\"e30ca493-d5d4-4c79-9ea0-2752edd701ef\"}]},\"type\":\"ConnectorPlacement.EquallySpacedConnector\",\"uuid\":\"a290fee4-a270-4f54-b8a3-7452b5039597\"}],\"packageUris\":[\"http://schema.mathworks.com/mf0/Connector/R2020b\"],\"version\":\"1.0\"}"
  Subsystem6 : Subsystem
      settings: PortSchema="{\"entries\":[{\"content\":{\"sides\":[{\"content\":{},\"type\":\"ConnectorPlacement.EquallySpacedRectSide\",\"uuid\":\"89586188-a7fa-42d8-902c-41f5e85746df\"},{\"content\":{\"connectorIds\":[\"Out1\"],\"side\":\"RIGHT\"},\"type\":\"ConnectorPlacement.EquallySpacedRectSide\",\"uuid\":\"d8c02237-7822-43ca-9dbf-595cafdf61ba\"},{\"content\":{\"connectorIds\":[\"LConn1\",\"Out2\"],\"side\":\"TOP\"},\"type\":\"ConnectorPlacement.EquallySpacedRectSide\",\"uuid\":\"69757e4c-b908-4056-b98e-0c667e12b99a\"},{\"content\":{\"connectorIds\":[\"RConn1\",\"In1\"],\"side\":\"BOTTOM\"},\"type\":\"ConnectorPlacement.EquallySpacedRectSide\",\"uuid\":\"e30ca493-d5d4-4c79-9ea0-2752edd701ef\"}]},\"type\":\"ConnectorPlacement.EquallySpacedConnector\",\"uuid\":\"a290fee4-a270-4f54-b8a3-7452b5039597\"}],\"packageUris\":[\"http://schema.mathworks.com/mf0/Connector/R2020b\"],\"version\":\"1.0\"}"
  Subsystem7 : Subsystem
      settings: PortSchema="{\"entries\":[{\"content\":{\"sides\":[{\"content\":{},\"type\":\"ConnectorPlacement.EquallySpacedRectSide\",\"uuid\":\"89586188-a7fa-42d8-902c-41f5e85746df\"},{\"content\":{\"connectorIds\":[\"Out1\"],\"side\":\"RIGHT\"},\"type\":\"ConnectorPlacement.EquallySpacedRectSide\",\"uuid\":\"d8c02237-7822-43ca-9dbf-595cafdf61ba\"},{\"content\":{\"connectorIds\":[\"LConn1\",\"Out2\"],\"side\":\"TOP\"},\"type\":\"ConnectorPlacement.EquallySpacedRectSide\",\"uuid\":\"69757e4c-b908-4056-b98e-0c667e12b99a\"},{\"content\":{\"connectorIds\":[\"RConn1\",\"In1\"],\"side\":\"BOTTOM\"},\"type\":\"ConnectorPlacement.EquallySpacedRectSide\",\"uuid\":\"e30ca493-d5d4-4c79-9ea0-2752edd701ef\"}]},\"type\":\"ConnectorPlacement.EquallySpacedConnector\",\"uuid\":\"a290fee4-a270-4f54-b8a3-7452b5039597\"}],\"packageUris\":[\"http://schema.mathworks.com/mf0/Connector/R2020b\"],\"version\":\"1.0\"}"
  To File1 : ToFile  Filename=sup_res
  wires:
  [v_ramp] -> Subsystem7/1(V_low)
  Constant/1 -> [i_conv]
  [v_ramp] -> Subsystem6/1(V_low)
  [i_conv] -> Controlled Current Source3/1
  [i_sup3] -> Mux6/5
  Subsystem7/2(i_supp) -> [i_sup3]
  Mux6/1 -> Scope/1, To File1/1
  Subsystem3/1(i_supp) -> [i_sup1]
  [i_conv] -> Controlled Current Source1/1
  Stair Generator3/1 -> [v_ramp]
  [i_conv] -> Mux6/1
  [i_sup2] -> Mux6/4
  [i_sup1] -> Mux6/3
  [i_conv] -> Controlled Current Source2/1
  Subsystem6/2(i_supp) -> [i_sup2]
  [v_ramp] -> Subsystem3/1(V_low)
  [v_ramp] -> Mux6/2
  Subsystem7/1(V_in) -> [v_in3]
  [v_in3] -> Mux6/8
  Subsystem1/1(i_supp) -> [i_sup4]
  [i_conv] -> Controlled Current Source4/1
  [v_ramp] -> Subsystem1/1(V_low)
  [i_sup4] -> Mux6/6
  Subsystem6/1(V_in) -> [v_in2]
  [v_in2] -> Mux6/7
  connections:
  Controlled Current Source3/RConn1 -- Subsystem7/LConn1
  Controlled Current Source3/LConn1 -- Subsystem7/RConn1
  Controlled Current Source2/RConn1 -- Subsystem6/LConn1
  Controlled Current Source2/LConn1 -- Subsystem6/RConn1
  Controlled Current Source1/RConn1 -- Subsystem3/LConn1
  Subsystem3/RConn1 -- Controlled Current Source1/LConn1
  Controlled Current Source4/RConn1 -- Subsystem1/LConn1
  Subsystem1/RConn1 -- Controlled Current Source4/LConn1

== system main_sim_mk15_pi/reject 0s ==
  In : Inport
  MATLAB Function : MATLAB Function  TreatAsAtomicUnit=on
  Out : Outport
  wires:
  MATLAB Function/1(y) -> Out/1
  In/1 -> MATLAB Function/1(u)

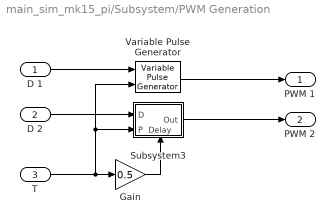
== system main_sim_mk15_pi/Subsystem/PWM Generation ==
  D 1 : Inport
  D 2 : Inport  Port=2
  T : Inport  Port=3
  Gain : Gain  Gain=0.5
  Subsystem3 : Subsystem
      settings: PortSchema="{\"entries\":[{\"content\":{\"sides\":[{\"content\":{\"connectorIds\":[\"In1\",\"In2\"]},\"type\":\"ConnectorPlacement.EquallySpacedRectSide\",\"uuid\":\"51b045c8-d819-4b7c-a29d-1a54f5fd995d\"},{\"content\":{\"connectorIds\":[\"Out1\"],\"side\":\"RIGHT\"},\"type\":\"ConnectorPlacement.EquallySpacedRectSide\",\"uuid\":\"9f0647dc-9c35-4883-9e64-6da00897cce8\"},{\"content\":{\"side\":\"TOP\"},\"type\":\"ConnectorPlacement.EquallySpacedRectSide\",\"uuid\":\"a4aa7abf-9a58-441d-bef7-3a2aafbde944\"},{\"content\":{\"connectorIds\":[\"In3\"],\"side\":\"BOTTOM\"},\"type\":\"ConnectorPlacement.EquallySpacedRectSide\",\"uuid\":\"95ada6aa-cdcb-4fa7-a4c9-da06f440da05\"}]},\"type\":\"ConnectorPlacement.EquallySpacedConnector\",\"uuid\":\"237ebc79-3794-4318-8db8-2d16dc313947\"}],\"packageUris\":[\"http://schema.mathworks.com/mf0/Connector/R2020b\"],\"version\":\"1.0\"}"
  Variable Pulse Generator : VariablePulseGenerator  SampleTime=0.1
  PWM 1 : Outport
  PWM 2 : Outport  Port=2
  wires:
  D 2/1 -> Subsystem3/1(D)
  Subsystem3/1(Out) -> PWM 2/1
  T/1 -> Gain/1, Subsystem3/2(P), Variable Pulse Generator/2
  Variable Pulse Generator/1 -> PWM 1/1
  D 1/1 -> Variable Pulse Generator/1
  Gain/1 -> Subsystem3/3(Delay)

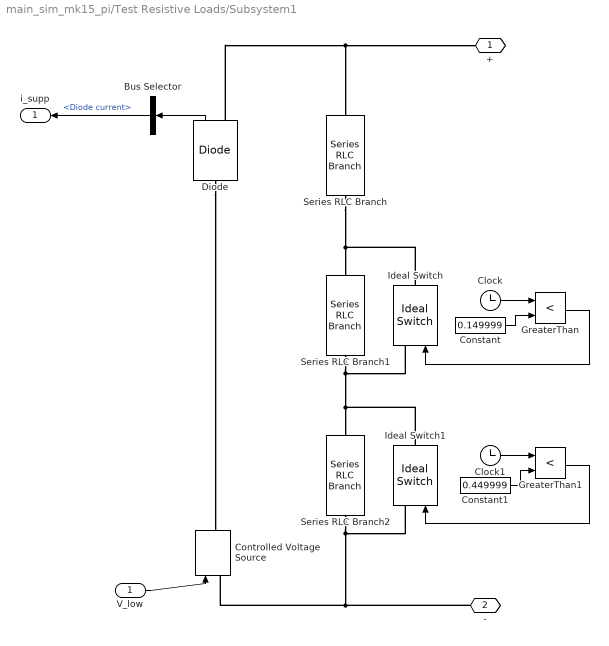
== system main_sim_mk15_pi/Test Resistive Loads/Subsystem1 ==
  V_low : Inport
  Bus Selector : BusSelector  OutputSignals=Diode current
  Clock : Clock
  Clock1 : Clock
  Constant : Constant  Value=0.149999
  Constant1 : Constant  Value=0.449999
  Controlled Voltage Source : spsControlledVoltageSourceLib/Controlled Voltage Source  Initialize=on  Source_Type=DC  Amplitude=40  Phase=0  Frequency=0  Measurements=None
  Diode : spsDiodeLib/Diode  Ron=0.001  Lon=0  Vf=0.01  IC=0  UseSnubber=0  Rs=500  Cs=250e-9  Measurements=on
  GreaterThan : RelationalOperator  Operator=<  OutDataTypeStr=boolean  RndMeth=Simplest  InputSameDT=off
  GreaterThan1 : RelationalOperator  Operator=<  OutDataTypeStr=boolean  RndMeth=Simplest  InputSameDT=off
  Ideal Switch : spsIdealSwitchLib/Ideal Switch  Ron=0.001  Lon=0  IC=0  Rs=1e5  Cs=inf  Measurements=off
  Ideal Switch1 : spsIdealSwitchLib/Ideal Switch  Ron=0.001  Lon=0  IC=0  Rs=1e5  Cs=inf  Measurements=off
  Series RLC Branch : spsSeriesRLCBranchLib/Series RLC Branch  LConnTagsString=__new0  RConnTagsString=__new0  BranchType=R  Resistance=0.32  Inductance=1e-9  SetiL0=off  InitialCurrent=0  Capacitance=1e-6  Setx0=off  InitialVoltage=0  Measurements=None
  Series RLC Branch1 : spsSeriesRLCBranchLib/Series RLC Branch  LConnTagsString=__new0  RConnTagsString=__new0  BranchType=R  Resistance=0.33  Inductance=1e-3  SetiL0=off  InitialCurrent=0  Capacitance=1e-6  Setx0=off  InitialVoltage=0  Measurements=None
  Series RLC Branch2 : spsSeriesRLCBranchLib/Series RLC Branch  LConnTagsString=__new0  RConnTagsString=__new0  BranchType=R  Resistance=0.5  Inductance=1e-3  SetiL0=off  InitialCurrent=0  Capacitance=1e-6  Setx0=off  InitialVoltage=0  Measurements=None
  + : PMIOPort  Side=Left
  - : PMIOPort  Port=2  Side=Right
  i_supp : Outport
  wires:
  Diode/1 -> Bus Selector/1
  Bus Selector/1 -> i_supp/1  "<Diode current>"
  V_low/1 -> Controlled Voltage Source/1
  Clock/1 -> GreaterThan/1
  Constant/1 -> GreaterThan/2
  GreaterThan/1 -> Ideal Switch/1
  Constant1/1 -> GreaterThan1/2
  Clock1/1 -> GreaterThan1/1
  GreaterThan1/1 -> Ideal Switch1/1
  connections:
  Diode/LConn1 -- Controlled Voltage Source/RConn1
  Ideal Switch/RConn1 -- Series RLC Branch/RConn1 -- Series RLC Branch1/LConn1
  Series RLC Branch1/RConn1 -- Series RLC Branch2/LConn1 -- Ideal Switch1/RConn1 -- Ideal Switch/LConn1
  Series RLC Branch2/RConn1 -- -/RConn1 -- Controlled Voltage Source/LConn1 -- Ideal Switch1/LConn1
  Diode/RConn1 -- Series RLC Branch/LConn1 -- +/RConn1

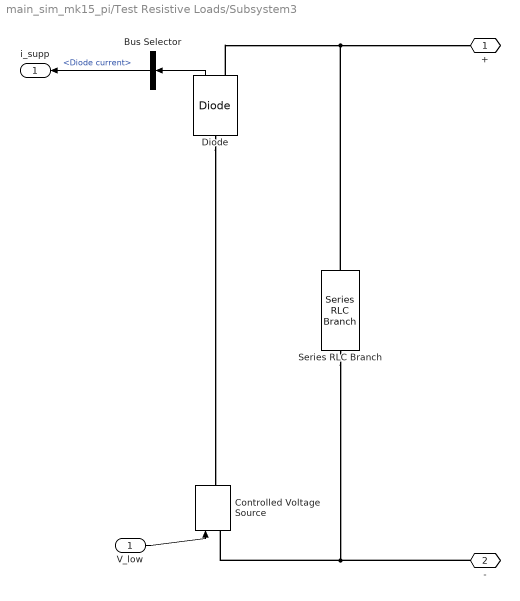
== system main_sim_mk15_pi/Test Resistive Loads/Subsystem3 ==
  V_low : Inport
  Bus Selector : BusSelector  OutputSignals=Diode current
  Controlled Voltage Source : spsControlledVoltageSourceLib/Controlled Voltage Source  Initialize=on  Source_Type=DC  Amplitude=40  Phase=0  Frequency=0  Measurements=None
  Diode : spsDiodeLib/Diode  Ron=0.001  Lon=0  Vf=0.01  IC=0  UseSnubber=0  Rs=500  Cs=250e-9  Measurements=on
  Series RLC Branch : spsSeriesRLCBranchLib/Series RLC Branch  LConnTagsString=__new0  RConnTagsString=__new0  BranchType=R  Resistance=0.32  Inductance=1e-3  SetiL0=off  InitialCurrent=0  Capacitance=1e-6  Setx0=off  InitialVoltage=0  Measurements=None
  + : PMIOPort  Side=Left
  - : PMIOPort  Port=2  Side=Right
  i_supp : Outport
  wires:
  Diode/1 -> Bus Selector/1
  Bus Selector/1 -> i_supp/1  "<Diode current>"
  V_low/1 -> Controlled Voltage Source/1
  connections:
  Diode/RConn1 -- Series RLC Branch/LConn1 -- +/RConn1
  Diode/LConn1 -- Controlled Voltage Source/RConn1
  -/RConn1 -- Controlled Voltage Source/LConn1 -- Series RLC Branch/RConn1

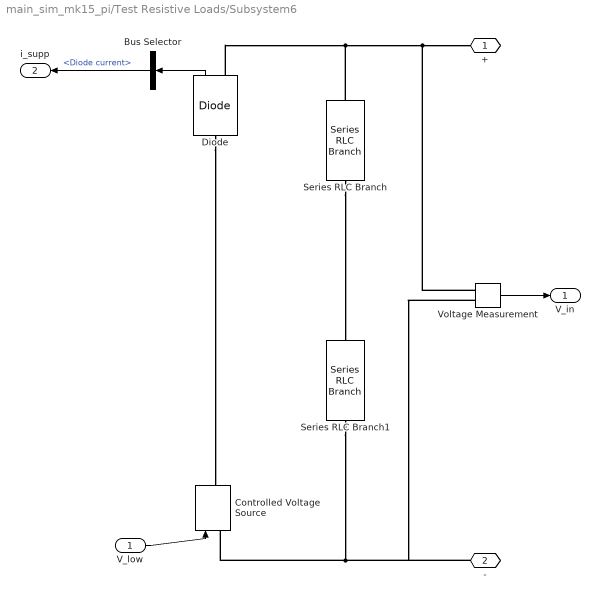
== system main_sim_mk15_pi/Test Resistive Loads/Subsystem6 ==
  V_low : Inport
  Bus Selector : BusSelector  OutputSignals=Diode current
  Controlled Voltage Source : spsControlledVoltageSourceLib/Controlled Voltage Source  Initialize=on  Source_Type=DC  Amplitude=40  Phase=0  Frequency=0  Measurements=None
  Diode : spsDiodeLib/Diode  Ron=0.001  Lon=0  Vf=0.01  IC=0  UseSnubber=0  Rs=500  Cs=250e-9  Measurements=on
  Series RLC Branch : spsSeriesRLCBranchLib/Series RLC Branch  LConnTagsString=__new0  RConnTagsString=__new0  BranchType=R  Resistance=0.32  Inductance=1e-3  SetiL0=off  InitialCurrent=0  Capacitance=1e-6  Setx0=off  InitialVoltage=0  Measurements=None
  Series RLC Branch1 : spsSeriesRLCBranchLib/Series RLC Branch  LConnTagsString=__new0  RConnTagsString=__new0  BranchType=R  Resistance=0.33  Inductance=1e-3  SetiL0=off  InitialCurrent=0  Capacitance=1e-6  Setx0=off  InitialVoltage=0  Measurements=None
  Voltage Measurement : spsVoltageMeasurementLib/Voltage Measurement  PhasorSimulation=off  OutputType=Complex  PSBequivalent=0
  + : PMIOPort  Side=Left
  - : PMIOPort  Port=2  Side=Right
  V_in : Outport
  i_supp : Outport  Port=2
  wires:
  Diode/1 -> Bus Selector/1
  Bus Selector/1 -> i_supp/1  "<Diode current>"
  V_low/1 -> Controlled Voltage Source/1
  Voltage Measurement/1 -> V_in/1
  connections:
  Diode/RConn1 -- Series RLC Branch/LConn1 -- Voltage Measurement/LConn1 -- +/RConn1
  Diode/LConn1 -- Controlled Voltage Source/RConn1
  Series RLC Branch/RConn1 -- Series RLC Branch1/LConn1
  Series RLC Branch1/RConn1 -- Voltage Measurement/LConn2 -- -/RConn1 -- Controlled Voltage Source/LConn1

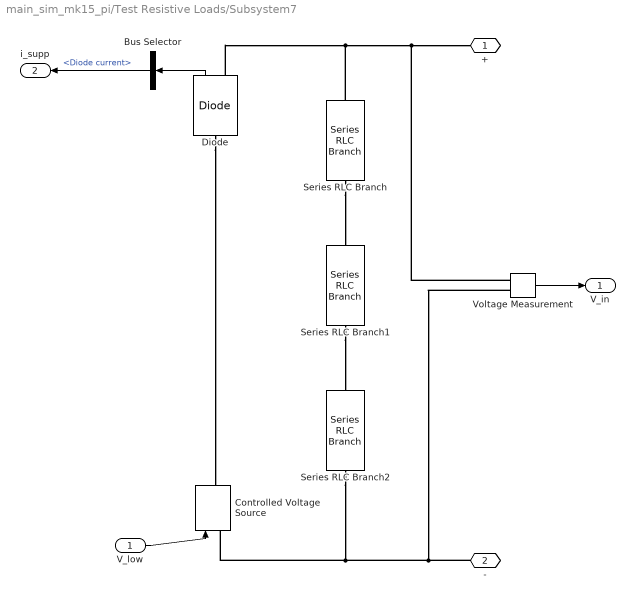
== system main_sim_mk15_pi/Test Resistive Loads/Subsystem7 ==
  V_low : Inport
  Bus Selector : BusSelector  OutputSignals=Diode current
  Controlled Voltage Source : spsControlledVoltageSourceLib/Controlled Voltage Source  Initialize=on  Source_Type=DC  Amplitude=40  Phase=0  Frequency=0  Measurements=None
  Diode : spsDiodeLib/Diode  Ron=0.001  Lon=0  Vf=0.01  IC=0  UseSnubber=0  Rs=500  Cs=250e-9  Measurements=on
  Series RLC Branch : spsSeriesRLCBranchLib/Series RLC Branch  LConnTagsString=__new0  RConnTagsString=__new0  BranchType=R  Resistance=0.32  Inductance=1e-3  SetiL0=off  InitialCurrent=0  Capacitance=1e-6  Setx0=off  InitialVoltage=0  Measurements=None
  Series RLC Branch1 : spsSeriesRLCBranchLib/Series RLC Branch  LConnTagsString=__new0  RConnTagsString=__new0  BranchType=R  Resistance=0.33  Inductance=1e-3  SetiL0=off  InitialCurrent=0  Capacitance=1e-6  Setx0=off  InitialVoltage=0  Measurements=None
  Series RLC Branch2 : spsSeriesRLCBranchLib/Series RLC Branch  LConnTagsString=__new0  RConnTagsString=__new0  BranchType=R  Resistance=0.5  Inductance=1e-3  SetiL0=off  InitialCurrent=0  Capacitance=1e-6  Setx0=off  InitialVoltage=0  Measurements=None
  Voltage Measurement : spsVoltageMeasurementLib/Voltage Measurement  PhasorSimulation=off  OutputType=Complex  PSBequivalent=0
  + : PMIOPort  Side=Left
  - : PMIOPort  Port=2  Side=Right
  V_in : Outport
  i_supp : Outport  Port=2
  wires:
  Diode/1 -> Bus Selector/1
  Bus Selector/1 -> i_supp/1  "<Diode current>"
  V_low/1 -> Controlled Voltage Source/1
  Voltage Measurement/1 -> V_in/1
  connections:
  Diode/RConn1 -- Series RLC Branch/LConn1 -- Voltage Measurement/LConn1 -- +/RConn1
  Diode/LConn1 -- Controlled Voltage Source/RConn1
  Series RLC Branch/RConn1 -- Series RLC Branch1/LConn1
  Series RLC Branch1/RConn1 -- Series RLC Branch2/LConn1
  -/RConn1 -- Voltage Measurement/LConn2 -- Controlled Voltage Source/LConn1 -- Series RLC Branch2/RConn1

== system main_sim_mk15_pi/Subsystem/PWM Generation/Subsystem3 ==
  D : Inport
  P : Inport  Port=2
  Delay : Inport  Port=3
  Clock1 : Clock
  GreaterThan : RelationalOperator  Operator=>  OutDataTypeStr=boolean  RndMeth=Simplest  InputSameDT=off
  Subsystem : Subsystem
  Out : Outport
  wires:
  Clock1/1 -> GreaterThan/1
  P/1 -> Subsystem/2(P)
  GreaterThan/1 -> Subsystem/Enable
  D/1 -> Subsystem/1(D)
  Delay/1 -> GreaterThan/2
  Subsystem/1(Out) -> Out/1

== system main_sim_mk15_pi/Subsystem/PWM Generation/Subsystem3/Subsystem ==
  D : Inport
  P : Inport  Port=2
  Enable : EnablePort
  Variable Pulse Generator1 : VariablePulseGenerator  AllowZeroPulseWidth=on  SampleTime=0.1
  Out : Outport
  wires:
  D/1 -> Variable Pulse Generator1/1
  Variable Pulse Generator1/1 -> Out/1
  P/1 -> Variable Pulse Generator1/2

== matlab function main_sim_mk15_pi/Subsystem/MATLAB Function ==
  data: pwm1 input; m1_p output; pwm2 input; mode input; enable_synch_mode input; m2_p output; m3_p output; m4_p output
function [m1_p,m2_p,m3_p,m4_p] = call_route_pcc_signals(pwm1,pwm2,mode,enable_synch_mode)

    [m1_p,m2_p,m3_p,m4_p] = route_pcc_signals(pwm1,pwm2,mode,enable_synch_mode);
end

== matlab function main_sim_mk15_pi/reject 0s/MATLAB Function ==
  data: u input; y output
function y = fcn(u)
if u==0
    y=0.001;
else 
    y=u;
end
y = u;

== matlab function main_sim_mk15_pi/Subsystem/MATLAB Function1 ==
  settings: updateMethod=DISCRETE
  data: i_dc_link input; duty1 output; v_dc_link input; v_sc input; i_ind_1 input; i_ind_2 input; clock input; stop_all output; mode output; i_ind_ref output; kp input; ki input
function [duty1,stop_all,mode,i_ind_ref]= call_central_cntrl(i_dc_link,v_dc_link,v_sc,i_ind_1,i_ind_2,clock,kp, ki)


[duty1,stop_all,mode,i_ind_ref]=central_cntrl(i_dc_link,v_dc_link,v_sc,i_ind_1,i_ind_2,clock,kp, ki);

== matlab function main_sim_mk15_pi/Interleaved, 2 Branches/MATLAB Function ==
  data: i_in input; eff output; p_in input; p_out input
function eff = eff_calc(i_in,p_in,p_out)

if i_in>=0
    eff=min(max(p_in/p_out,0),1);
else
    eff=min(max(p_out/p_in,0),1);
end
